simulink model "design"  (R2022b)
settings: Solver=VariableStepAuto  StartTime=0.0  StopTime=10.0  RelTol=1e-3
settings Model: Creator=Lyn  LastModifiedBy=Lyn

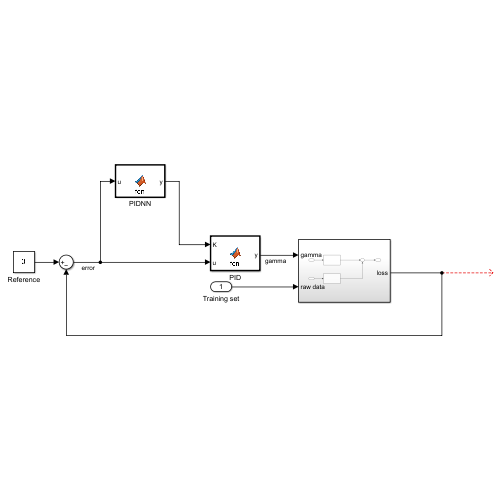
[thumbnail: Simulink's stored preview of the top-level diagram]
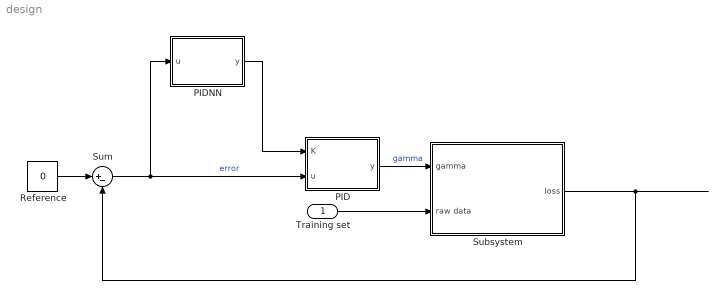
== system design ==
  Training set : Inport
  PID : MATLAB Function  TreatAsAtomicUnit=on
  PIDNN : MATLAB Function  TreatAsAtomicUnit=on
  Reference : Constant  Value=0
  Subsystem : Subsystem
  Sum : Sum  Inputs=|+-
  wires:
  Sum/1 -> PIDNN/1(u), PID/2(u)  "error"
  Reference/1 -> Sum/1
  Subsystem/1(loss) -> Sum/2
  PID/1(y) -> Subsystem/1(gamma)  "gamma"
  Training set/1 -> Subsystem/2(raw data)
  PIDNN/1(y) -> PID/1(K)

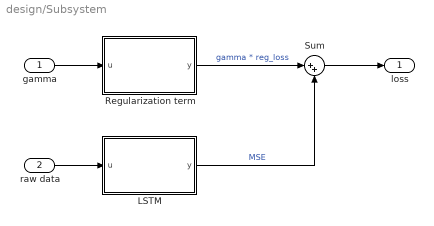
== system design/Subsystem ==
  gamma : Inport
  raw data : Inport  Port=2
  LSTM : MATLAB Function  TreatAsAtomicUnit=on
  Regularization term : MATLAB Function  TreatAsAtomicUnit=on
  Sum : Sum  Inputs=|++
  loss : Outport
  wires:
  raw data/1 -> LSTM/1(u)
  LSTM/1(y) -> Sum/2  "MSE"
  gamma/1 -> Regularization term/1(u)
  Regularization term/1(y) -> Sum/1  "gamma * reg_loss"
  Sum/1 -> loss/1

== matlab function design/Subsystem/LSTM ==
  data: u input; y output
function y = fcn(u)

y = u;

== matlab function design/Subsystem/Regularization term ==
  data: u input; y output
function y = fcn(u)

y = u;

== matlab function design/PIDNN ==
  data: u input; y output
function y = fcn(u)

y = u;

== matlab function design/PID ==
  data: K input; u input; y output
function y = fcn(K, u)

y = u;
